simulink model "acc_with_sensor"  (R2021b)
(part 7 of 9)

  Constant8 : Constant  Value="[0\t1.3813498\t2.7674625\t4.1505508\t5.5305071\t6.9074359\t8.2817230\t9.6630182\t11.067275\t12.500264\t13.966639\t15.462024\t16.969576\t18.483765\t19.999269\t21.513163\t23.024817\t24.534275\t26.041573\t27.546707\t29.049662\t30.550430\t32.049004\t33.545383\t35.039570\t36.531555\t38.021347\t39.508942\t40.994343\t42.477551\t43.958569\t45.437397\t46.914040\t48.388500\t49.860779\t51.330921\t52.798996\t54.265007\t55.728954\t57.190838\t58.650661\t60.108429\t61.564140\t63.017799\t64.469406\t65.918968\t67.366478\t68.811951\t70.255379\t71.696770\t73.136124\t74.573441\t76.008728\t77.441978\t78.873207\t80.302406\t81.729584\t83.154739\t84.577873\t85.998985\t87.418091\t88.835175\t90.250252\t91.663315\t93.074379\t94.483429\t95.890480\t97.295532\t98.698586\t100.09964\t101.49870\t102.89576\t104.29083\t105.68392\t107.07509\t108.46471\t109.85322\t111.24086\t112.62796\t114.01488\t115.40186\t116.78905\t118.17657\t119.56448\t120.95287\t122.34178\t123.73123\t125.12125\t126.51182\t127.90295\t129.29463\t130.68683\t132.07953\t133.47269\t134.86629\t136.26028\t137.65466\t139.04936\t140.44438\t141.83966\t143.23518\t144.63092\t146.02686\t147.42294\t148.81920\t150.21556\t151.61206\t153.00864\t154.40532\t155.80208\t157.19891\t158.59583\t159.99278\t161.38982\t162.78693\t164.18408\t165.58130\t166.97859\t168.37595\t169.77338\t171.17087\t172.56844\t173.96608\t175.36382\t176.76163\t178.15952\t179.55750\t180.95557\t182.35373\t183.75200\t185.15034\t186.54880\t187.94734\t189.34599\t190.74475\t192.14360\t193.54256\t194.94162\t196.34079\t197.74005\t199.13942\t200.53889\t201.93848\t203.33817\t204.73795\t206.13785\t207.53784\t208.93794\t210.33815\t211.73846\t213.13887\t214.53938\t215.94000\t217.34073\t218.74155\t220.14247\t221.54350\t222.94464\t224.34587\t225.74721\t227.14865\t228.55020\t229.95184\t231.35359\t232.75543\t234.15739\t235.55945\t236.96161\t238.36386\t239.76622\t241.16870\t242.57126\t243.97394\t245.37671\t246.77959\t248.18257\t249.58565\t250.98882\t252.39198\t253.79515\t255.19833\t256.60150\t258.00467\t259.40787\t260.81104\t262.21423\t263.61743\t265.02063\t266.42380\t267.82700\t269.23022\t270.63342\t272.03662\t273.43982\t274.84302\t276.24625\t277.64944\t279.05267\t280.45587\t281.85910\t283.26230\t284.66553\t286.06873\t287.47195\t288.87515\t290.27838\t291.68158\t293.08481\t294.48801\t295.89124\t297.29443\t298.69766\t300.10086\t301.50409\t302.90729\t304.31052\t305.71371\t307.11694\t308.52014\t309.92337\t311.32657\t312.72977\t314.13300\t315.53619\t316.93942\t318.34262\t319.74585\t321.14905\t322.55228\t323.95547\t325.35867\t326.76190\t328.16510\t329.56833\t330.97153\t332.37476\t333.77795\t335.18115\t336.58438\t337.98758\t339.39081\t340.79401\t342.19724\t343.60043\t345.00363\t346.40686\t347.81006\t349.21329\t350.61649\t352.01971\t353.42291\t354.82611\t356.22934\t357.63254\t359.03577\t360.43896\t361.84219\t363.24539\t364.64862\t366.05182\t367.44269\t368.83173\t370.22079\t371.60986\t372.99896\t374.38806\t375.77719\t377.16629\t378.55539\t379.94449\t381.33356\t382.72263\t384.11166\t385.50070\t386.88971\t388.27869\t389.66769\t391.05664\t392.44562\t393.83453\t395.22348\t396.61240\t398.00131\t399.39020\t400.77911\t402.16800\t403.55688\t404.94577\t406.33466\t407.72351\t409.11240\t410.50125\t411.89014\t413.27902\t414.66788\t416.05676\t417.44562\t418.83450\t420.22339\t421.61224\t423.00113\t424.39001\t425.77890\t427.16779\t428.55667\t429.94556\t431.33444\t432.72333\t434.11221\t435.50110\t436.88998\t438.27887\t439.66776\t441.05664\t442.44553\t443.83441\t445.22333\t446.61221\t448.00110\t449.38998\t450.77887\t452.16776\t453.55664\t454.94556\t456.33444\t457.72333\t459.11221\t460.50110\t461.88998\t463.27887\t464.66779\t466.05667\t467.44556\t468.83444\t470.22333\t471.61221\t473.00110\t474.38998\t475.77887\t477.16779\t478.55667\t479.94556\t481.33444\t482.72333\t484.11221\t485.50110\t486.88998\t488.27887\t489.66779\t491.05667\t492.44556\t493.83444\t495.22333\t496.61221\t498.00110\t499.38998\t500.77887\t502.16779\t503.55667\t504.94556\t506.33444\t507.72333\t509.11221\t510.50110\t511.88998\t513.27887\t514.66779\t516.05664\t517.44556\t518.83441\t520.22333\t521.61224\t523.00110\t524.39001\t525.77887\t527.16779\t528.55664\t529.94556\t531.33441\t532.72333\t534.11224\t535.50110\t536.89001\t538.27887\t539.66779\t541.05664\t542.44556\t543.83441\t545.22333\t546.61224\t548.00110\t549.39001\t550.77887\t552.16779\t553.55664\t554.94556\t556.33441\t557.72333\t559.11224\t560.50110\t561.89001\t563.27887\t564.66779\t566.05664\t567.44550\t568.83429\t570.22290\t571.61151\t572.99994\t574.38831\t575.77661\t577.16479\t578.55286\t579.94086\t581.32874\t582.71655\t584.10425\t585.49182\t586.87933\t588.26672\t589.65405\t591.04126\t592.42841\t593.81543\t595.20233\t596.58917\t597.97589\t599.36255\t600.74908\t602.13556\t603.52191\t604.90814\t606.29431\t607.68036\t609.06635\t610.45221\t611.83801\t613.22369\t614.60925\t615.99475\t617.38019\t618.76544\t620.15070\t621.53577\t622.92084\t624.30573\t625.69055\t627.07532\t628.45996\t629.84448\t631.22894\t632.61328\t633.99756\t635.38171\t636.76581\t638.14978\t639.53363\t640.91742\t642.30115\t643.68475\t645.06824\t646.45166\t647.83496\t649.21820\t650.60132\t651.98438\t653.36731\t654.75018\t656.13293\t657.51556\t658.89813\t660.28064\t661.66302\t663.04529\t664.42749\t665.80957\t667.19159\t668.57355\t669.95532\t671.33710\t672.71869\t674.10022\t675.48169\t676.86304\t678.24432\t679.62549\t681.00659\t682.38757\t683.76843\t685.14923\t686.52997\t687.91058\t689.29108\t690.67151\t692.05182\t693.43207\t694.81226\t696.19232\t697.57227\t698.95215\t700.33191\t701.71161\t703.09125\t704.47070\t705.85016\t707.22949\t708.60870\t709.98785\t711.36688\t712.74585\t714.12469\t715.50348\t716.88214\t718.26074\t719.63922\t721.01764\t722.39594\t723.77417\t725.15234\t726.53033\t727.90833\t729.28619\t730.66394\t732.04163\t733.41919\t734.79669\t736.17413\t737.55139\t738.92865\t740.30579\t741.68280\t743.05975\t744.43665\t745.81342\t747.19006\t748.56665\t749.94318\t751.31958\t752.69586\t754.07214\t755.44824\t756.82428\t758.20026\t759.57611\t760.95190\t762.32758\t763.70319\t765.07867\t766.45410\t767.82953\t769.20490\t770.58026\t771.95569\t773.33105\t774.70648\t776.08185\t777.45728\t778.83270\t780.20807\t781.58350\t782.95892\t784.33435\t785.70978\t787.08521\t788.46063\t789.83606\t791.21149\t792.58691\t793.96234\t795.33777\t796.71320\t798.08862\t799.46405\t800.83948\t802.21490\t803.59033\t804.96576\t806.34119\t807.71661\t809.09204\t810.46747\t811.84290\t813.21832\t814.59375\t815.96918\t817.34460\t818.72009\t820.09552\t821.47095\t822.84637\t824.22180\t825.59723\t826.97266\t828.34808\t829.72351\t831.09894\t832.47437\t833.84979\t835.22522\t836.60065\t837.97607\t839.35150\t840.72693\t842.10236\t843.47778\t844.85321\t846.22864\t847.60406\t848.97949\t850.35492\t851.73035\t853.10577\t854.48120\t855.85663\t857.23206\t858.60748\t859.98291\t861.35834\t862.73376\t864.10919\t865.48462\t866.86005\t868.23547\t869.61090\t870.98633\t872.36176\t873.73718\t875.11261\t876.48804\t877.86346\t879.23895\t880.61438\t881.98981\t883.37396\t884.76294\t886.15198\t887.54108\t888.93018\t890.31927\t891.70837\t893.09747\t894.48657\t895.87561\t897.26471\t898.65375\t900.04279\t901.43182\t902.82086\t904.20984\t905.59882\t906.98779\t908.37677\t909.76569\t911.15460\t912.54352\t913.93243\t915.32135\t916.71027\t918.09912\t919.48804\t920.87689\t922.26581\t923.65466\t925.04352\t926.43243\t927.82129\t929.21014\t930.59906\t931.98792\t933.37677\t934.76569\t936.15454\t937.54340\t938.93231\t940.32117\t941.71002\t943.09894\t944.48779\t945.87671\t947.26556\t948.65448\t950.04333\t951.43225\t952.82111\t954.21002\t955.59894\t956.98779\t958.37671\t959.76556\t961.15448\t962.54333\t963.93225\t965.32117\t966.71002\t968.09894\t969.48779\t970.87671\t972.26556\t973.65448\t975.04340\t976.43225\t977.82117\t979.21002\t980.59894\t981.98779\t983.37671\t984.76556\t986.15448\t987.54340\t988.93225\t990.32117\t991.71002\t993.09894\t994.48779\t995.87671\t997.26556\t998.65448\t1000.0434\t1001.4323\t1002.8212\t1004.2100\t1005.5989\t1006.9878\t1008.3767\t1009.7656\t1011.1545\t1012.5434\t1013.9323\t1015.3212\t1016.7100\t1018.0989\t1019.4878\t1020.8767\t1022.2656\t1023.6545\t1025.0433\t1026.4323\t1027.8212\t1029.2101\t1030.5989\t1031.9878\t1033.3767\t1034.7656\t1036.1545\t1037.5433\t1038.9323\t1040.3212\t1041.7101\t1043.0989\t1044.4878\t1045.8767\t1047.2656\t1048.6545\t1050.0433\t1051.4323\t1052.8212\t1054.2101\t1055.5989\t1056.9878\t1058.3767\t1059.7656\t1061.1545\t1062.5433\t1063.9323\t1065.3212\t1066.7101\t1068.0989\t1069.4878\t1070.8767\t1072.2656\t1073.6545\t1075.0433\t1076.4323\t1077.8212\t1079.2101\t1080.5989\t1081.9878\t1083.3767\t1084.7656\t1086.1545\t1087.5433\t1088.9323\t1090.3212\t1091.7101\t1093.0989\t1094.4878\t1095.8767\t1097.2656\t1098.6545\t1100.0433\t1101.4323\t1102.8212\t1104.2101\t1105.5989\t1106.9878\t1108.3767\t1109.7656\t1111.1545\t1112.5433\t1113.9323\t1115.3212\t1116.7101\t1118.0989\t1119.4878\t1120.8767\t1122.2656\t1123.6545\t1125.0433\t1126.4323\t1127.8212\t1129.2101\t1130.5989\t1131.9878\t1133.3767\t1134.7656\t1136.1545\t1137.5433\t1138.9323\t1140.3212\t1141.7101\t1143.0989\t1144.4878\t1145.8767\t1147.2656\t1148.6545\t1150.0433\t1151.4323\t1152.8212\t1154.2101\t1155.5989\t1156.9878\t1158.3767\t1159.7656\t1161.1545\t1162.5433\t1163.9323\t1165.3212\t1166.7101\t1168.0989\t1169.4878\t1170.8767\t1172.2656\t1173.6545\t1175.0433\t1176.4323\t1177.8212\t1179.2101\t1180.5989\t1181.9878\t1183.3767\t1184.7656\t1186.1545\t1187.5433\t1188.9323\t1190.3212\t1191.7101\t1193.0989\t1194.4878\t1195.8767\t1197.2656\t1198.6545\t1200.0433\t1201.4323\t1202.8212\t1204.2101\t1205.5989\t1206.9878\t1208.3767\t1209.7656\t1211.1545\t1212.5433\t1213.9323\t1215.3212\t1216.7101\t1218.0989\t1219.4878\t1220.8767\t1222.2656\t1223.6545\t1225.0433\t1226.4323\t1227.8212\t1229.2101\t1230.5989\t1231.9878\t1233.3767\t1234.7656\t1236.1545\t1237.5433\t1238.9323\t1240.3212\t1241.7101\t1243.0989\t1244.4878\t1245.8767\t1247.2656\t1248.6545\t1250.0433\t1251.4323\t1252.8212\t1254.2101\t1255.5989\t1256.9878\t1258.3767\t1259.7656\t1261.1545\t1262.5433\t1263.9323\t1265.3212\t1266.7101\t1268.0989\t1269.4878\t1270.8767\t1272.2656\t1273.6545\t1275.0433\t1276.4323\t1277.8212\t1279.2101\t1280.5989\t1281.9878\t1283.3767\t1284.7656\t1286.1545\t1287.5433\t1288.9323\t1290.3212\t1291.7101\t1293.0989\t1294.4878\t1295.8767\t1297.2656\t1298.6545\t1300.0433\t1301.4323\t1302.8212\t1304.2101\t1305.5989\t1306.9878\t1308.3767\t1309.7656\t1311.1545\t1312.5433\t1313.9323\t1315.3212\t1316.7101\t1318.0989\t1319.4878\t1320.8767\t1322.2656\t1323.6545\t1325.0433\t1326.4323\t1327.8212\t1329.2101\t1330.5989\t1331.9878\t1333.3767\t1334.7656\t1336.1545\t1337.5433\t1338.9323\t1340.3212\t1341.7101\t1343.0989\t1344.4878\t1345.8767\t1347.2656\t1348.6545\t1350.0433\t1351.4323\t1352.8212\t1354.2101\t1355.5989\t1356.9878\t1358.3767\t1359.7656\t1361.1545\t1362.5433\t1363.9323\t1365.3212\t1366.7101\t1368.0989\t1369.4878\t1370.8767\t1372.2656\t1373.6545\t1375.0433\t1376.4323\t1377.8212\t1379.2101\t1380.5989\t1381.9878\t1383.3767\t1384.7656\t1386.1545\t1387.5433\t1388.9323\t1390.3212\t1391.7101\t1393.0989\t1394.4878\t1395.8767\t1397.2656\t1398.6545\t1400.0433\t1401.4323\t1402.8212\t1404.2101\t1405.5989\t1406.9878\t1408.3767\t1409.7656\t1411.1545\t1412.5433\t1413.9323\t1415.3212\t1416.7101\t1418.0989\t1419.4878\t1420.8767\t1422.2656\t1423.6545\t1425.0433\t1426.4323\t1427.8212\t1429.2101\t1430.5989\t1431.9878\t1433.3767\t1434.7656\t1436.1545\t1437.5433\t1438.9323\t1440.3212\t1441.7101\t1443.0989\t1444.4878\t1445.8767\t1447.2656\t1448.6545\t1450.0433\t1451.4323\t1452.8212\t1454.2101\t1455.5989\t1456.9878\t1458.3767\t1459.7656\t1461.1545\t1462.5433\t1463.9323\t1465.3212\t1466.7101\t1468.0989\t1469.4878\t1470.8767\t1472.2656\t1473.6545\t1475.0433\t1476.4323\t1477.8212\t1479.2101\t1480.5989\t1481.9878\t1483.3767\t1484.7656\t1486.1545\t1487.5433\t1488.9323\t1490.3212\t1491.7101\t1493.0989\t1494.4878\t1495.8767\t1497.2656\t1498.6545\t1500.0433\t1501.4323\t1502.8212\t1504.2101\t1505.5989\t1506.9878\t1508.3767\t1509.7656\t1511.1545\t1512.5433\t1513.9323\t1515.3212\t1516.7101\t1518.0989\t1519.4878\t1520.8767\t1522.2656\t1523.6545\t1525.0433\t1526.4323\t1527.8212\t1529.2101\t1530.5989\t1531.9878\t1533.3767\t1534.7656\t1536.1545\t1537.5433\t1538.9323\t1540.3212\t1541.7101\t1543.0989\t1544.4878\t1545.8767\t1547.2656\t1548.6545\t1550.0433\t1551.4323\t1552.8212\t1554.2101\t1555.5989\t1556.9878\t1558.3767\t1559.7656\t1561.1545\t1562.5433\t1563.9323\t1565.3212\t1566.7101\t1568.0989\t1569.4878\t1570.8767\t1572.2656\t1573.6545\t1575.0433\t1576.4323\t1577.8212\t1579.2101\t1580.5989\t1581.9878\t1583.3767\t1584.7656\t1586.1545\t1587.5433\t1588.9323\t1590.3212\t1591.7101\t1593.0989\t1594.4878\t1595.8767\t1597.2656\t1598.6545\t1600.0433\t1601.4323\t1602.8212\t1604.2101\t1605.5989\t1606.9878\t1608.3767\t1609.7656\t1611.1545\t1612.5433\t1613.9323\t1615.3212\t1616.7101\t1618.0989\t1619.4878\t1620.8767\t1622.2656\t1623.6545\t1625.0433\t1626.4323\t1627.8212\t1629.2101\t1630.5989\t1631.9878\t1633.3767\t1634.7656\t1636.1545\t1637.5433\t1638.9323\t1640.3212\t1641.7101\t1643.0989\t1644.4878\t1645.8767\t1647.2656\t1648.6545\t1650.0433\t1651.4323\t1652.8212\t1654.2101\t1655.5989\t1656.9878\t1658.3767\t1659.7656\t1661.1545\t1662.5433\t1663.9323\t1665.3212\t1666.7101\t1668.0989\t1669.4878\t1670.8767\t1672.2656\t1673.6545\t1675.0433\t1676.4323\t1677.8212\t1679.2101\t1680.5989\t1681.9878\t1683.3767\t1684.7656\t1686.1545\t1687.5433\t1688.9323\t1690.3212\t1691.7101\t1693.0989\t1694.4878\t1695.8767\t1697.2656\t1698.6545\t1700.0433\t1701.4323\t1702.8212\t1704.2101\t1705.5989\t1706.9878\t1708.3767\t1709.7656\t1711.1545\t1712.5433\t1713.9323\t1715.3212\t1716.7101\t1718.0989\t1719.4878\t1720.8767\t1722.2656\t1723.6545\t1725.0433\t1726.4323\t1727.8212\t1729.2101\t1730.5989\t1731.9878\t1733.3767\t1734.7656\t1736.1545\t1737.5433\t1738.9323\t1740.3212\t1741.7101\t1743.0989\t1744.4878\t1745.8767\t1747.2656\t1748.6545\t1750.0433\t1751.4323\t1752.8212\t1754.2101\t1755.5989\t1756.9878\t1758.3767\t1759.7656\t1761.1545\t1762.5433\t1763.9323\t1765.3212\t1766.7101\t1768.0989\t1769.4878\t1770.8767\t1772.2656\t1773.6545\t1775.0433\t1776.4323\t1777.8212\t1779.2101\t1780.5989\t1781.9878\t1783.3767\t1784.7656\t1786.1545\t1787.5433\t1788.9323\t1790.3212\t1791.7101\t1793.0989\t1794.4878\t1795.8767\t1797.2656\t1798.6545\t1800.0433\t1801.4323\t1802.8212\t1804.2101\t1805.5989\t1806.9878\t1808.3767\t1809.7656\t1811.1545\t1812.5433\t1813.9323\t1815.3212\t1816.7101\t1818.0989\t1819.4878\t1820.8767\t1822.2656\t1823.6545\t1825.0433\t1826.4323\t1827.8212\t1829.2101\t1830.5989\t1831.9878\t1833.3767\t1834.7656\t1836.1545\t1837.5433\t1838.9323\t1840.3212\t1841.7101\t1843.0989\t1844.4878\t1845.8767\t1847.2656\t1848.6545\t1850.0433\t1851.4323\t1852.8212\t1854.2101\t1855.5989\t1856.9878\t1858.3767\t1859.7656\t1861.1545\t1862.5433\t1863.9323\t1865.3212\t1866.7101\t1868.0989\t1869.4878\t1870.8767\t1872.2656\t1873.6545\t1875.0433\t1876.4323\t1877.8212\t1879.2101\t1880.5989\t1881.9878\t1883.3767\t1884.7656\t1886.1545\t1887.5433\t1888.9323\t1890.3212\t1891.7101\t1893.0989\t1894.4878\t1895.8767\t1897.2656\t1898.6545\t1900.0433\t1901.4323\t1902.8212\t1904.2101\t1905.5989\t1906.9878\t1908.3767\t1909.7656\t1911.1545\t1912.5433\t1913.9323\t1915.3212\t1916.7101\t1918.0989\t1919.4878\t1920.8767\t1922.2656\t1923.6545\t1925.0433\t1926.4323\t1927.8212\t1929.2101\t1930.5989\t1931.9878\t1933.3767\t1934.7656\t1936.1545\t1937.5433\t1938.9323\t1940.3212\t1941.7101\t1943.0989\t1944.4878\t1945.8767\t1947.2656\t1948.6545\t1950.0433\t1951.4323\t1952.8212\t1954.2101\t1955.5989\t1956.9878\t1958.3767\t1959.7656\t1961.1545\t1962.5433\t1963.9323\t1965.3212\t1966.7101\t1968.0989\t1969.4878\t1970.8767\t1972.2656\t1973.6545\t1975.0433\t1976.4323\t1977.8212\t1979.2101\t1980.5989\t1981.9878\t1983.3767\t1984.7656\t1986.1545\t1987.5433\t1988.9323\t1990.3212\t1991.7101\t1993.0989\t1994.4878\t1995.8767\t1997.2656\t1998.6545\t2000.0433\t2001.4323\t2002.8212\t2004.2101\t2005.5989\t2006.9878\t2008.3767\t2009.7656\t2011.1545\t2012.5433\t2013.9323\t2015.3212\t2016.7101\t2018.0989\t2019.4878\t2020.8767\t2022.2656\t2023.6545\t2025.0433\t2026.4323\t2027.8212\t2029.2101\t2030.5989\t2031.9878\t2033.3767\t2034.7656\t2036.1545\t2037.5433\t2038.9323\t2040.3212\t2041.7101\t2043.0989\t2044.4878\t2045.8767\t2047.2656\t2048.6545\t2050.0435\t2051.4324\t2052.8210\t2054.2100\t2055.5989\t2056.9878\t2058.3767\t2059.7656\t2061.1545\t2062.5435\t2063.9324\t2065.3210\t2066.7100\t2068.0989\t2069.4878\t2070.8767\t2072.2656\t2073.6545\t2075.0435\t2076.4324\t2077.8210\t2079.2100\t2080.5989\t2081.9878\t2083.3767\t2084.7656\t2086.1545\t2087.5435\t2088.9324\t2090.3210\t2091.7100\t2093.0989\t2094.4878\t2095.8767\t2097.2656\t2098.6545\t2100.0435\t2101.4324\t2102.8210\t2104.2100\t2105.5989\t2106.9878\t2108.3767\t2109.7656\t2111.1545\t2112.5435\t2113.9324\t2115.3210\t2116.7100\t2118.0989\t2119.4878\t2120.8767\t2122.2656\t2123.6545\t2125.0435\t2126.4324\t2127.8210\t2129.2100\t2130.5989\t2131.9878\t2133.3767\t2134.7656\t2136.1545\t2137.5435\t2138.9324\t2140.3210\t2141.7100\t2143.0989\t2144.4878\t2145.8767\t2147.2656\t2148.6545\t2150.0435\t2151.4324\t2152.8210\t2154.2100\t2155.5989\t2156.9878\t2158.3767\t2159.7656\t2161.1545\t2162.5435\t2163.9324\t2165.3210\t2166.7100\t2168.0989\t2169.4878\t2170.8767\t2172.2656\t2173.6545\t2175.0435\t2176.4324\t2177.8210\t2179.2100\t2180.5989\t2181.9878\t2183.3767\t2184.7656\t2186.1545\t2187.5435\t2188.9324\t2190.3210\t2191.7100\t2193.0989\t2194.4878\t2195.8767\t2197.2656\t2198.6545\t2200.0435\t2201.4324\t2202.8210\t2204.2100\t2205.5989\t2206.9878\t2208.3767\t2209.7656\t2211.1545\t2212.5435\t2213.9324\t2215.3210\t2216.7100\t2218.0989\t2219.4878\t2220.8767\t2222.2656\t2223.6545\t2225.0435\t2226.4324\t2227.8210\t2229.2100\t2230.5989\t2231.9878\t2233.3767\t2234.7656\t2236.1545\t2237.5435\t2238.9324\t2240.3210\t2241.7100\t2243.0989\t2244.4878\t2245.8767\t2247.2656\t2248.6545\t2250.0435\t2251.4324\t2252.8210\t2254.2100\t2255.5989\t2256.9878\t2258.3767\t2259.7656\t2261.1545\t2262.5435\t2263.9324\t2265.3210\t2266.7100\t2268.0989\t2269.4878\t2270.8767\t2272.2656\t2273.6545\t2275.0435\t2276.4324\t2277.8210\t2279.2100\t2280.5989\t2281.9878\t2283.3767\t2284.7656\t2286.1545\t2287.5435\t2288.9324\t2290.3210\t2291.7100\t2293.0989\t2294.4878\t2295.8767\t2297.2656\t2298.6545\t2300.0435\t2301.4324\t2302.8210\t2304.2100\t2305.5989\t2306.9878\t2308.3767\t2309.7656\t2311.1545\t2312.5435\t2313.9324\t2315.3210\t2316.7100\t2318.0989\t2319.4878\t2320.8767\t2322.2656\t2323.6545\t2325.0435\t2326.4324\t2327.8210\t2329.2100\t2330.5989\t2331.9878\t2333.3767\t2334.7656\t2336.1545\t2337.5435\t2338.9324\t2340.3210\t2341.7100\t2343.0989\t2344.4878\t2345.8767\t2347.2656\t2348.6545\t2350.0435\t2351.4324\t2352.8210\t2354.2100\t2355.5989\t2356.9878\t2358.3767\t2359.7656\t2361.1545\t2362.5435\t2363.9324\t2365.3210\t2366.7100\t2368.0989\t2369.4878\t2370.8767\t2372.2656\t2373.6545\t2375.0435\t2376.4324\t2377.8210\t2379.2100\t2380.5989\t2381.9878\t2383.3767\t2384.7656\t2386.1545\t2387.5435\t2388.9324\t2390.3210\t2391.7100\t2393.0989\t2394.4878\t2395.8767\t2397.2656\t2398.6545\t2400.0435\t2401.4324\t2402.8210\t2404.2100\t2405.5989\t2406.9878\t2408.3767\t2409.7656\t2411.1545\t2412.5435\t2413.9324\t2415.3210\t2416.7100\t2418.0989\t2419.4878\t2420.8767\t2422.2656\t2423.6545\t2425.0435\t2426.4324\t2427.8210\t2429.2100\t2430.5989\t2431.9878\t2433.3767\t2434.7656\t2436.1545\t2437.5435\t2438.9324\t2440.3210\t2441.7100\t2443.0989\t2444.4878\t2445.8767\t2447.2656\t2448.6545\t2450.0435\t2451.4324\t2452.8210\t2454.2100\t2455.5989\t2456.9878\t2458.3767\t2459.7656\t2461.1545\t2462.5435\t2463.9324\t2465.3210\t2466.7100\t2468.0989\t2469.4878\t2470.8767\t2472.2656\t2473.6545\t2475.0435\t2476.4324\t2477.8210\t2479.2100\t2480.5989\t2481.9878\t2483.3767\t2484.7656\t2486.1545\t2487.5435\t2488.9324\t2490.3210\t2491.7100\t2493.0989\t2494.4878\t2495.8767\t2497.2656\t2498.6545\t2500.0435\t2501.4324\t2502.8210\t2504.2100\t2505.5989\t2506.9878\t2508.3767\t2509.7656\t2511.1545\t2512.5435\t2513.9324\t2515.3210\t2516.7100\t2518.0989\t2519.4878\t2520.8767\t2522.2656\t2523.6545\t2525.0435\t2526.4324\t2527.8210\t2529.2100\t2530.5989\t2531.9878\t2533.3767\t2534.7656\t2536.1545\t2537.5435\t2538.9324\t2540.3210\t2541.7100\t2543.0989\t2544.4878\t2545.8767\t2547.2656\t2548.6545\t2550.0435\t2551.4324\t2552.8210\t2554.2100\t2555.5989\t2556.9878\t2558.3767\t2559.7656\t2561.1545\t2562.5435\t2563.9324\t2565.3210\t2566.7100\t2568.0989\t2569.4878\t2570.8767\t2572.2656\t2573.6545\t2575.0435\t2576.4324\t2577.8210\t2579.2100\t2580.5989\t2581.9878\t2583.3767\t2584.7656\t2586.1545\t2587.5435\t2588.9324\t2590.3210\t2591.7100\t2593.0989\t2594.4878\t2595.8767\t2597.2656\t2598.6545\t2600.0435\t2601.4324\t2602.8210\t2604.2100\t2605.5989\t2606.9878\t2608.3767\t2609.7656\t2611.1545\t2612.5435\t2613.9324\t2615.3210\t2616.7100\t2618.0989\t2619.4878\t2620.8767\t2622.2656\t2623.6545\t2625.0435\t2626.4324\t2627.8210\t2629.2100\t2630.5989\t2631.9878\t2633.3767\t2634.7656\t2636.1545\t2637.5435\t2638.9324\t2640.3210\t2641.7100\t2643.0989\t2644.4878\t2645.8767\t2647.2656\t2648.6545\t2650.0435\t2651.4324\t2652.8210\t2654.2100\t2655.5989\t2656.9878\t2658.3767\t2659.7656\t2661.1545\t2662.5435\t2663.9324\t2665.3210\t2666.7100\t2668.0989\t2669.4878\t2670.8767\t2672.2656\t2673.6545\t2675.0435\t2676.4324\t2677.8210\t2679.2100\t2680.5989\t2681.9878\t2683.3767\t2684.7656\t2686.1545\t2687.5435\t2688.9324\t2690.3210\t2691.7100\t2693.0989\t2694.4878\t2695.8767\t2697.2656\t2698.6545\t2700.0435\t2701.4324\t2702.8210\t2704.2100\t2705.5989\t2706.9878\t2708.3767\t2709.7656\t2711.1545\t2712.5435\t2713.9324\t2715.3210\t2716.7100\t2718.0989\t2719.4878\t2720.8767\t2722.2656\t2723.6545\t2725.0435\t2726.4324\t2727.8210\t2729.2100\t2730.5989\t2731.9878\t2733.3767\t2734.7656\t2736.1545\t2737.5435\t2738.9324\t2740.3210\t2741.7100\t2743.0989\t2744.4878\t2745.8767\t2747.2656\t2748.6545\t2750.0435\t2751.4324\t2752.8210\t2754.2100\t2755.5989\t2756.9878\t2758.3767\t2759.7656\t2761.1545\t2762.5435\t2763.9324\t2765.3210\t2766.7100\t2768.0989\t2769.4878\t2770.8767\t2772.2656\t2773.6545\t2775.0435\t2776.4324\t2777.8210\t2779.2100\t2780.5989\t2781.9878\t2783.3767\t2784.7656\t2786.1545\t2787.5435\t2788.9324\t2790.3210\t2791.7100\t2793.0989\t2794.4878\t2795.8767\t2797.2656\t2798.6545\t2800.0435\t2801.4324\t2802.8210\t2804.2100\t2805.5989\t2806.9878\t2808.3767\t2809.7656\t2811.1545\t2812.5435\t2813.9324\t2815.3210\t2816.7100\t2818.0989\t2819.4878\t2820.8767\t2822.2656\t2823.6545\t2825.0435\t2826.4324\t2827.8210\t2829.2100\t2830.5989\t2831.9878\t2833.3767\t2834.7656\t2836.1545\t2837.5435\t2838.9324\t2840.3210\t2841.7100\t2843.0989\t2844.4878\t2845.8767\t2847.2656\t2848.6545\t2850.0435\t2851.4324\t2852.8210\t2854.2100\t2855.5989\t2856.9878\t2858.3767\t2859.7656\t2861.1545\t2862.5435\t2863.9324\t2865.3210\t2885.9412\t2885.9512\t2885.9612\t2885.9712\t2885.9812\t2885.9912\t2886.0012\t2886.0112\t2886.0212\t2886.0313\t2886.0413\t2886.0513\t2886.0610\t2886.0710\t2886.0811\t2886.0911\t2886.1011\t2886.1111\t2886.1211\t2886.1311\t2886.1411\t2886.1511\t2886.1611\t2886.1711\t2886.1812\t2886.1912\t2886.2012\t2886.2112\t2886.2212\t2886.2312\t2886.2412\t2886.2512\t2886.2612\t2886.2712\t2886.2813\t2886.2913\t2886.3013\t2886.3110\t2886.3210\t2886.3311\t2886.3411\t2886.3511\t2886.3611\t2886.3711\t2886.3811\t2886.3911\t2886.4011\t2886.4111\t2886.4211\t2886.4312\t2886.4412\t2886.4512\t2886.4612\t2886.4712\t2886.4812\t2886.4912\t2886.5012\t2886.5112\t2886.5212\t2886.5313\t2886.5413\t2886.5513\t2886.5610\t2886.5710\t2886.5811\t2886.5911\t2886.6011\t2886.6111\t2886.6211\t2886.6311\t2886.6411\t2886.6511\t2886.6611\t2886.6711\t2886.6812\t2886.6912\t2886.7012\t2886.7112\t2886.7212\t2886.7312\t2886.7412\t2886.7512\t2886.7612\t2886.7712\t2886.7813\t2886.7913\t2886.8013\t2886.8110\t2886.8210\t2886.8311\t2886.8411\t2886.8511\t2886.8611\t2886.8711\t2886.8811\t2886.8911\t2886.9011\t2886.9111\t2886.9211\t2886.9312\t2886.9412\t2886.9512\t2886.9612\t2886.9712\t2886.9812\t2886.9912\t2887.0012\t2887.0112\t2887.0212\t2887.0313\t2887.0413\t2887.0513\t2887.0610\t2887.0710\t2887.0811\t2887.0911\t2887.1011\t2887.1111\t2887.1211\t2887.1311\t2887.1411\t2887.1511\t2887.1611\t2887.1711\t2887.1812\t2887.1912\t2887.2012\t2887.2112\t2887.2212\t2887.2312\t2887.2412\t2887.2512\t2887.2612\t2887.2712\t2887.2813\t2887.2913\t2887.3013\t2887.3110\t2887.3210\t2887.3311\t2887.3411\t2887.3511\t2887.3611\t2887.3711\t2887.3811\t2887.3911\t2887.4011\t2887.4111\t2887.4211\t2887.4312\t2887.4412\t2887.4512\t2887.4612\t2887.4712\t2887.4812\t2887.4912\t2887.5012\t2887.5112\t2887.5212\t2887.5313\t2887.5413\t2887.5513\t2887.5610\t2887.5710\t2887.5811\t2887.5911\t2887.6011\t2887.6111\t2887.6211\t2887.6311\t2887.6411\t2887.6511\t2887.6611\t2887.6711\t2887.6812\t2887.6912\t2887.7012\t2887.7112\t2887.7212\t2887.7312\t2887.7412\t2887.7512\t2887.7612\t2887.7712\t2887.7813\t2887.7913\t2887.8013\t2887.8110\t2887.8210\t2887.8311\t2887.8411\t2887.8511\t2887.8611\t2887.8711\t2887.8811\t2887.8911\t2887.9011\t2887.9111\t2887.9211\t2887.9312\t2887.9412\t2887.9512\t2887.9612\t2887.9712\t2887.9812\t2887.9912\t2888.0012\t2888.0112\t2888.0212\t2888.0313\t2888.0413\t2888.0513\t2888.0610\t2888.0710\t2888.0811\t2888.0911\t2888.1011\t2888.1111\t2888.1211\t2888.1311\t2888.1411\t2888.1511\t2888.1611\t2888.1711\t2888.1812\t2888.1912\t2888.2012\t2888.2112\t2888.2212\t2888.2312\t2888.2412\t2888.2512\t2888.2612\t2888.2712\t2888.2813\t2888.2913\t2888.3013\t2888.3110\t2888.3210\t2888.3311\t2888.3411\t2888.3511\t2888.3611\t2888.3711\t2888.3811\t2888.3911\t2888.4011\t2888.4111\t2888.4211\t2888.4312\t2888.4412\t2888.4512\t2888.4612\t2888.4712\t2888.4812\t2888.4912\t2888.5012\t2888.5112\t2888.5212\t2888.5313\t2888.5413\t2888.5513\t2888.5610\t2888.5710\t2888.5811\t2888.5911\t2888.6011\t2888.6111\t2888.6211\t2888.6311\t2888.6411\t2888.6511\t2888.6611\t2888.6711\t2888.6812\t2888.6912\t2888.7012\t2888.7112\t2888.7212\t2888.7312\t2888.7412\t2888.7512\t2888.7612\t2888.7712\t2888.7813\t2888.7913\t2888.8013\t2888.8110\t2888.8210\t2888.8311\t2888.8411\t2888.8511\t2888.8611\t2888.8711\t2888.8811\t2888.8911\t2888.9011\t2888.9111\t2888.9211\t2888.9312\t2888.9412\t2888.9512\t2888.9612\t2888.9712\t2888.9812\t2888.9912\t2889.0012\t2889.0112\t2889.0212\t2889.0313\t2889.0413\t2889.0513\t2889.0610\t2889.0710\t2889.0811\t2889.0911\t2889.1011\t2889.1111\t2889.1211\t2889.1311\t2889.1411\t2889.1511\t2889.1611\t2889.1711\t2889.1812\t2889.1912\t2889.2012\t2889.2112\t2889.2212\t2889.2312\t2889.2412\t2889.2512\t2889.2612\t2889.2712\t2889.2813\t2889.2913\t2889.3013\t2889.3110\t2889.3210\t2889.3311\t2889.3411\t2889.3511\t2889.3611\t2889.3711\t2889.3811\t2889.3911\t2889.4011\t2889.4111\t2889.4211\t2889.4312\t2889.4412\t2889.4512\t2889.4612\t2889.4712\t2889.4812\t2889.4912\t2889.5012\t2889.5112\t2889.5212\t2889.5313\t2889.5413\t2889.5513\t2889.5610\t2889.5710\t2889.5811\t2889.5911\t2889.6011\t2889.6111\t2889.6211\t2889.6311\t2889.6411\t2889.6511\t2889.6611\t2889.6711\t2889.6812\t2889.6912\t2889.7012\t2889.7112\t2889.7212\t2889.7312\t2889.7412\t2889.7512\t2889.7612\t2889.7712\t2889.7813\t2889.7913\t2889.8013\t2889.8110\t2889.8210\t2889.8311\t2889.8411\t2889.8511\t2889.8611\t2889.8711\t2889.8811\t2889.8911\t2889.9011\t2889.9111\t2889.9211\t2889.9312\t2889.9412\t2889.9512\t2889.9612\t2889.9712\t2889.9812\t2889.9912\t2890.0012\t2890.0112\t2890.0212\t2890.0313\t2890.0413\t2890.0513\t2890.0610\t2890.0710\t2890.0811\t2890.0911\t2890.1011\t2890.1111\t2890.1211\t2890.1311\t2890.1411\t2890.1511\t2890.1611\t2890.1711\t2890.1812\t2890.1912\t2890.2012\t2890.2112\t2890.2212\t2890.2312\t2890.2412\t2890.2512\t2890.2612\t2890.2712\t2890.2813\t2890.2913\t2890.3013\t2890.3110\t2890.3210\t2890.3311\t2890.3411\t2890.3511\t2890.3611\t2890.3711\t2890.3811\t2890.3911\t2890.4011\t2890.4111\t2890.4211\t2890.4312\t2890.4412\t2890.4512\t2890.4612\t2890.4712\t2890.4812\t2890.4912\t2890.5012\t2890.5112\t2890.5212\t2890.5313\t2890.5413\t2890.5513\t2890.5610\t2890.5710\t2890.5811\t2890.5911\t2890.6011\t2890.6111\t2890.6211\t2890.6311\t2890.6411\t2890.6511\t2890.6611\t2890.6711\t2890.6812\t2890.6912\t2890.7012\t2890.7112\t2890.7212\t2890.7312\t2890.7412\t2890.7512\t2890.7612\t2890.7712\t2890.7813\t2890.7913\t2890.8013\t2890.8110\t2890.8210\t2890.8311\t2890.8411\t2890.8511\t2890.8611\t2890.8711\t2890.8811\t2890.8911\t2890.9011\t2890.9111\t2890.9211\t2890.9312\t2890.9412\t2890.9512\t2890.9612\t2890.9712\t2890.9812\t2890.9912\t2891.0012\t2891.0112\t2891.0212\t2891.0313\t2891.0413\t2891.0513\t2891.0610\t2891.0710\t2891.0811\t2891.0911\t2891.1011\t2891.1111\t2891.1211\t2891.1311\t2891.1411\t2891.1511\t2891.1611\t2891.1711\t2891.1812\t2891.1912\t2891.2012\t2891.2112\t2891.2212\t2891.2312\t2891.2412\t2891.2512\t2891.2612\t2891.2712\t2891.2813\t2891.2913\t2891.3013\t2891.3110\t2891.3210\t2891.3311\t2891.3411\t2891.3511\t2891.3611\t2891.3711\t2891.3811\t2891.3911\t2891.4011\t2891.4111\t2891.4211\t2891.4312\t2891.4412\t2891.4512\t2891.4612\t2891.4712\t2891.4812\t2891.4912\t2891.5012\t2891.5112\t2891.5212\t2891.5313\t2891.5413\t2891.5513\t2891.5610\t2891.5710\t2891.5811\t2891.5911\t2891.6011\t2891.6111\t2891.6211\t2891.6311\t2891.6411\t2891.6511\t2891.6611\t2891.6711\t2891.6812\t2891.6912\t2891.7012\t2891.7112\t2891.7212\t2891.7312\t2891.7412\t2891.7512\t2891.7612\t2891.7712\t2891.7813\t2891.7913\t2891.8013\t2891.8110\t2891.8210\t2891.8311\t2891.8411\t2891.8511\t2891.8611\t2891.8711\t2891.8811\t2891.8911\t2891.9011\t2891.9111\t2891.9211\t2891.9312\t2891.9412\t2891.9512\t2891.9612\t2891.9712\t2891.9812\t2891.9912\t2892.0012\t2892.0112\t2892.0212\t2892.0313\t2892.0413\t2892.0513\t2892.0610\t2892.0710\t2892.0811\t2892.0911\t2892.1011\t2892.1111\t2892.1211\t2892.1311\t2892.1411\t2892.1511\t2892.1611\t2892.1711\t2892.1812\t2892.1912\t2892.2012\t2892.2112\t2892.2212\t2892.2312\t2892.2412\t2892.2512\t2892.2612\t2892.2712\t2892.2813\t2892.2913\t2892.3013\t2892.3110\t2892.3210\t2892.3311\t2892.3411\t2892.3511\t2892.3611\t2892.3711\t2892.3811\t2892.3911\t2892.4011\t2892.4111\t2892.4211\t2892.4312\t2892.4412\t2892.4512\t2892.4612\t2892.4712\t2892.4812\t2892.4912\t2892.5012\t2892.5112\t2892.5212\t2892.5313\t2892.5413\t2892.5513\t2892.5610\t2892.5710\t2892.5811\t2892.5911\t2892.6011\t2892.6111\t2892.6211\t2892.6311\t2892.6411\t2892.6511\t2892.6611\t2892.6711\t2892.6812\t2892.6912\t2892.7012\t2892.7112\t2892.7212\t2892.7312\t2892.7412\t2892.7512\t2892.7612\t2892.7712\t2892.7813\t2892.7913\t2892.8013\t2892.8110\t2892.8210\t2892.8311\t2892.8411\t2892.8511\t2892.8611\t2892.8711\t2892.8811\t2892.8911\t2892.9011\t2892.9111\t2892.9211\t2892.9312\t2892.9412\t2892.9512\t2892.9612\t2892.9712\t2892.9812\t2892.9912\t2893.0012\t2893.0112\t2893.0212\t2893.0313\t2893.0413\t2893.0513\t2893.0610\t2893.0710\t2893.0811\t2893.0911\t2893.1011\t2893.1111\t2893.1211\t2893.1311\t2893.1411\t2893.1511\t2893.1611\t2893.1711\t2893.1812\t2893.1912\t2893.2012\t2893.2112\t2893.2212\t2893.2312\t2893.2412\t2893.2512\t2893.2612\t2893.2712\t2893.2813\t2893.2913\t2893.3013\t2893.3110\t2893.3210\t2893.3311\t2893.3411\t2893.3511\t2893.3611\t2893.3711\t2893.3811\t2893.3911\t2893.4011\t2893.4111\t2893.4211\t2893.4312\t2893.4412\t2893.4512\t2893.4612\t2893.4712\t2893.4812\t2893.4912\t2893.5012\t2893.5112\t2893.5212\t2893.5313\t2893.5413\t2893.5513\t2893.5610\t2893.5710\t2893.5811\t2893.5911\t2893.6011\t2893.6111\t2893.6211\t2893.6311\t2893.6411\t2893.6511\t2893.6611\t2893.6711\t2893.6812\t2893.6912\t2893.7012\t2893.7112\t2893.7212\t2893.7312\t2893.7412\t2893.7512\t2893.7612\t2893.7712\t2893.7813\t2893.7913\t2893.8013\t2893.8110\t2893.8210\t2893.8311\t2893.8411\t2893.8511\t2893.8611\t2893.8711\t2893.8811\t2893.8911\t2893.9011\t2893.9111\t2893.9211\t2893.9312\t2893.9412\t2893.9512\t2893.9612\t2893.9712\t2893.9812\t2893.9912\t2894.0012\t2894.0112\t2894.0212\t2894.0313\t2894.0413\t2894.0513\t2894.0610\t2894.0710\t2894.0811\t2894.0911\t2894.1011\t2894.1111\t2894.1211\t2894.1311\t2894.1411\t2894.1511\t2894.1611\t2894.1711\t2894.1812\t2894.1912\t2894.2012\t2894.2112\t2894.2212\t2894.2312\t2894.2412\t2894.2512\t2894.2612\t2894.2712\t2894.2813\t2894.2913\t2894.3013\t2894.3110\t2894.3210\t2894.3311\t2894.3411\t2894.3511\t2894.3611\t2894.3711\t2894.3811\t2894.3911\t2894.4011\t2894.4111\t2894.4211\t2894.4312\t2894.4412\t2894.4512\t2894.4612\t2894.4712\t2894.4812\t2894.4912\t2894.5012\t2894.5112\t2894.5212\t2894.5313\t2894.5413\t2894.5513\t2894.5610\t2894.5710\t2894.5811\t2894.5911\t2894.6011\t2894.6111\t2894.6211\t2894.6311\t2894.6411\t2894.6511\t2894.6611\t2894.6711\t2894.6812\t2894.6912\t2894.7012\t2894.7112\t2894.7212\t2894.7312\t2894.7412\t2894.7512\t2894.7612\t2894.7712\t2894.7813\t2894.7913\t2894.8013\t2894.8110\t2894.8210\t2894.8311\t2894.8411\t2894.8511\t2894.8611\t2894.8711\t2894.8811\t2894.8911\t2894.9011\t2894.9111\t2894.9211\t2894.9312\t2894.9412\t2894.9512\t2894.9612\t2894.9712\t2894.9812\t2894.9912\t2895.0012\t2895.0112\t2895.0212\t2895.0313\t2895.0413\t2895.0513\t2895.0610\t2895.0710\t2895.0811\t2895.0911\t2895.1011\t2895.1111\t2895.1211\t2895.1311\t2895.1411\t2895.1511\t2895.1611\t2895.1711\t2895.1812\t2895.1912\t2895.2012\t2895.2112\t2895.2212\t2895.2312\t2895.2412\t2895.2512\t2895.2612\t2895.2712\t2895.2813\t2895.2913\t2895.3013\t2895.3110\t2895.3210]'"  SampleTime=T
  Constant9 : Constant  Value=3  SampleTime=T
  Multiport Switch1 : MultiPortSwitch
  Multiport Switch2 : MultiPortSwitch
  Multiport Switch6 : MultiPortSwitch
  X_path : Outport
  s_path : Outport  Port=2
  Y_path : Outport  Port=3
  wires:
  Constant8/1 -> Multiport Switch1/4  "Clothoid_S_Turn"
  Constant7/1 -> Multiport Switch1/3  "4-Lane Section w/ Environment"
  Constant6/1 -> Multiport Switch2/4  "Clothoid_S_Turn"
  Constant5/1 -> Multiport Switch2/3  "4-Lane Section w/ Environment"
  Constant4/1 -> Multiport Switch2/2  "Straight_East_into_curve"
  Constant3/1 -> Multiport Switch1/2  "Straight_East_into_curve"
  Constant2/1 -> Multiport Switch6/4  "Clothoid_S_Turn"
  Constant1/1 -> Multiport Switch6/3  "4-Lane Section w/ Environment"
  Constant/1 -> Multiport Switch6/2  "Straight_East_into_curve"
  Constant9/1 -> Multiport Switch6/1, Multiport Switch2/1, Multiport Switch1/1
  Multiport Switch6/1 -> X_path/1
  Multiport Switch1/1 -> s_path/1
  Multiport Switch2/1 -> Y_path/1
